simulink model "System_Modell"  (R2018a)
settings: Solver=FixedStepAuto  StartTime=0.0  StopTime=inf  FixedStep=1/f  RelTol=1e-3
values from neighbouring files (symbols this model uses):
  f = 10000    [System_Init.m]
(part 7 of 8)

== matlab function System_Modell/Motor_3/MotionSM_1/MATLAB Function ==
  data: status input double size=1; excute_signal output boolean size=1; message_to_send output double size=2; data_received input double size=2; ZZP_wait data_store_memory size=1; AP data_store_memory; ZZP data_store_memory
%data_received / message_to_send = [cmd, ZZP]
%cmd:  1...setP, 2...getP, 3...excP

function [excute_signal, message_to_send] = message_analysis(status, data_received)

global ZZP_wait
global AP
global ZZP

excute_signal = false;

cmd = data_received(1);
message_to_send = [0, 0]';

switch cmd
    case 1      % setP
        excute_signal = false;
        if ((status >= 1) && (status <= 3))
            ZZP_wait = data_received(2);
            message_to_send = [2, ZZP_wait]';   % getP
        end
        
    case 3      % excP
        excute_signal = true;
        if ((ZZP == AP) && (status == 2) && (ZZP~=ZZP_wait))
            ZZP = ZZP_wait;
        end
end
end

== matlab function System_Modell/Motor_3/MotionSM_1/Motor/MATLAB Function ==
  settings: updateMethod=DISCRETE
  data: status_Motor output boolean size=1; Motor_control_signal input double size=1; parameter input double size=4; v input double size=1; a output double size=1; direction output double size=1; AP data_store_memory; ZZP data_store_memory
function [status_Motor, a, direction]= Motor(Motor_control_signal, parameter, v)

%delta_T = parameter(1);
a_max = abs(parameter(2));
v_max = abs(parameter(3));
s0 = parameter(4);
direction = 0;
a = 0;

s_a = 0.5 * v_max * v_max / a_max;
a_bremsen = 100000;     % 100 m/s^2

global AP
global ZZP

switch Motor_control_signal
    case {-1, 0}            %Error & Off
        if v > 0
            a = -a_bremsen;
            direction = 1;
        elseif v < 0
            a = a_bremsen;
            direction = -1;
        else
            a = 0;
            direction = 0;
        end
             
    case 1                  %Init
        if (AP > 0)
            direction = s0;
            if ((ZZP - AP) < (-s_a)) && (v > (-v_max))
                a = -a_max;
            elseif ((ZZP - AP) >= (-s_a)) && (ZZP < AP) && (v < 0)
                a = a_max;
            else
                a = 0;
            end
        else
            a = 0;
            AP = 0;
        end
        
    case 2                  %Stop
        if (v > 0)
            a = -a_max;
            direction = 1;
        elseif (v < 0)
            a = a_max;
            direction = -1;
        else
            a = 0;
            direction = 0;
        end
        
    case 3                  %run
        direction = s0;
        if (s0 > 0)   %forward
            %v_control(2) = s0;
            if ((ZZP - AP) > s_a) && (v < v_max)
                a = a_max;
            elseif ((ZZP - AP) <= s_a) && (ZZP > AP) && (v > 0)
                a = -a_max;
            else
                a = 0;
            end
        end
        if (s0 < 0)    %backward
            if ((ZZP - AP) < (-s_a)) && (v > (-v_max))
                a = -a_max;
            elseif ((ZZP - AP) >= (-s_a)) && (ZZP < AP) && (v < 0)
                a = a_max;
            else
                a = 0;
            end
        end
end
        
%status_Motor: false...Stopped, true...Running
if (a == 0) && (v == 0)
    status_Motor = false;
else
    status_Motor = true;
end

end

== matlab function System_Modell/Motor_3/MotionSM_1/Motor/MATLAB Function1 ==
  settings: updateMethod=DISCRETE
  data: V output; v input; direction input double size=1; AP data_store_memory; ZZP data_store_memory
function V = v_conrol(v, direction)

global AP
global ZZP

if direction > 0
    if ((v < 0) || (AP >= ZZP))
        V = 0;
    else
        V = v;
    end
elseif direction < 0
    if v > 0 || (AP <= ZZP)
        V = 0;
    else
        V = v;
    end
else
    V = 0;
end
end

== matlab function System_Modell/Motor_3/MotionSM_1/Motor/MATLAB Function2 ==
  settings: updateMethod=DISCRETE
  data: s input; s_old input; S output; direction input double size=1; AP data_store_memory; ZZP data_store_memory
function S = s_control(s, s_old, direction)

global AP
global ZZP

if direction > 0
    if (AP + s - s_old) < ZZP
        S = s;
        AP = AP + s - s_old;
    else
        S = s_old;
        AP = ZZP;
    end
elseif direction < 0
    if (AP + s - s_old) > ZZP
        S = s;
        AP = AP + s - s_old;
    else
        S = s_old;
        AP = ZZP;
    end
else
    S = s_old;
end

end

== matlab function System_Modell/Motor_3/Schnittstelle_0/Add_to_Send_Buffer ==
  data: Send_Buffer_1 data_store_memory; Send_Buffer_2 data_store_memory; Address data_store_memory; status input; lenS_1 input; lenS_2 input; to_send_signal input; to_send_package input; Address_1 data_store_memory; Address_2 data_store_memory; Handshake_1 data_store_memory; Handshake_2 data_store_memory; Filter data_store_memory; De_1 data_store_memory; De_2 data_store_memory; De_sum_1 data_store_memory; De_sum_2 data_store_memory
% Name: add_to_Send_Buffer
% Funktionalitäten
% Handshake-Message einfügen, wenn Status==1
% Delay-caculation-Message einfügen, wenn Status==2
% Sum-Delay-caculation-Message einfügen, wemm Status==3
% Nachrichten, die der Host senden möchte, einfügen, wenn Status==4

function add_to_Send_Buffer(status, lenS_1, lenS_2, to_send_signal, to_send_package)

global Send_Buffer_1
global Send_Buffer_2
global Address
global Address_1
global Address_2
global Handshake_1
global Handshake_2
global Filter
global De_1
global De_2
global De_sum_1
global De_sum_2

switch status
    case -2                         % Error Signal einrichten
        Filter(1,7) = 1;
    case 1                          % Handshake
        if((Filter(1,1) == 0) && ~Handshake_1)              % 103 not sent yet || Handshake_1 not finish yet
            check_1 = check_X(103, Address, Send_Buffer_1);          % check if there is a 103-Message in Send_Buffer_1
            if ~check_1
                Send_Buffer_1(lenS_1:lenS_1+7) = [Address, 0, 103, zeros(1,4), 102];
                Filter(1,1) = 1;                            % to remember, if 103 ist sent
            end
        end
        if((Filter(1,2) == 0) && ~Handshake_2)
            check_2 = check_X(103, Address, Send_Buffer_2);
            if ~check_2
                Send_Buffer_2(lenS_2:lenS_2+7) = [Address, 0, 103, zeros(1,4), 102];
                Filter(1,2) = 1;
            end
        end

        
    case 2                          % Delay time caculation
        if((Filter(1,3) == 0 ) && (De_1 <= 0))              % 105 not sent || De_1 not caculated yet
            check_1 = check_X(105, Address, Send_Buffer_1);
            if ~check_1
                Send_Buffer_1(lenS_1:lenS_1+7) = [Address, Address_2, 105, zeros(1,4), 102];
                Filter(1,3) = 1;
            end
        end
        if((Filter(1,4) == 0 ) && (De_2 <= 0))
            check_2 = check_X(105, Address, Send_Buffer_2);
            if ~check_2
                Send_Buffer_2(lenS_2:lenS_2+7) = [Address, Address_1, 105, zeros(1,4), 102];
                Filter(1,4) = 1;
            end
        end
        
    case 3                          % Sum_Delay caculation
        if((Filter(1,5) == 0 ) && (De_sum_1 <= 0))          % 107 not sent || De_sum_1 not caculated yet
            check_1 = check_X(107, Address, Send_Buffer_1);
            if ~check_1
                Send_Buffer_1(lenS_1:lenS_1+7) = [Address, Address, 107, zeros(1,4), 102];
                Filter(1,5) = 1;
            end
        end
        if((Filter(1,6) == 0 ) && (De_sum_2 <= 0))
            check_2 = check_X(107, Address, Send_Buffer_2);
            if ~check_2
                Send_Buffer_2(lenS_2:lenS_2+7) = [Address, Address, 107, zeros(1,4), 102];
                Filter(1,6) = 1;
            end
        end
        
    case 4                          % normal communication
        if to_send_signal
            check_1 = check_Y(to_send_package, Send_Buffer_1);
            check_2 = check_Y(to_send_package, Send_Buffer_2);
            if ~check_1
                Send_Buffer_1(lenS_1:lenS_1+7) = [to_send_package, 102];
            end
            if ~check_2
                Send_Buffer_2(lenS_2:lenS_2+7) = [to_send_package, 102];
            end
        end
end

end

function y = check_X(CMD, adr, Data)          % y: boolean; x: double, [1x100];

x = find(Data==CMD);
y = ~isempty(x);
if y
    y = y && (Data(1,x(1)-2) == adr);
end

end

function y = check_Y(data, Data)          % y: boolean; data: double, [1x6];

x = find(Data==data(3));        % CMD
y = ~isempty(x);
if y
    for i=1:length(x)
        if(isequal(Data(x(i)-2:x(i)+3),data(1:6)))
            y = true;
            break
        else
            y = false;
        end
    end
end

end

== matlab function System_Modell/Motor_3/Schnittstelle_0/Global_Var_Length ==
  data: len_Send_Buffer_1 output double size=1; len_Send_Buffer_2 output double size=1; len_Recv_Buffer output double size=1; len_Filter output double size=1; Send_Buffer_1 data_store_memory; Send_Buffer_2 data_store_memory; Recv_Buffer data_store_memory; Filter data_store_memory
% genutzte Länge der globale Variablen berechnen

function [len_Send_Buffer_1, len_Send_Buffer_2, len_Recv_Buffer, len_Filter] = Length
global Send_Buffer_1
global Send_Buffer_2
global Recv_Buffer
global Filter

a1 = find(Send_Buffer_1==102,1);
len_Send_Buffer_1 = a1(1);
a2 = find(Send_Buffer_2==102,1);
len_Send_Buffer_2 = a2(1);

len_Recv_Buffer = min(find(Recv_Buffer==0,150))-1;
len_Filter = min(find(Filter(2:20)==0,150));

end

== matlab function System_Modell/Motor_3/Schnittstelle_0/Recv_1 ==
  data: status input double size=1; clock input double size=1; lenS_1 input; lenS_2 input; lenR input; Rx_1_signal input boolean size=1; Rx_1_data input double size=[1 100]; recv_signal_1 output boolean; recv_package_1 output double size=[1 98]; Send_Buffer_1 data_store_memory; Send_Buffer_2 data_store_memory; T_send_1 data_store_memory; T_recv_1 data_store_memory; De_1 data_store_memory; De_sum_1 data_store_memory; Address data_store_memory; Recv_Buffer data_store_memory; Address_2 data_store_memory; Address_1 data_store_memory; De_sum_2 data_store_memory; Handshake_1 data_store_memory; De_2 data_store_memory; Handshake_2 data_store_memory; T_recv_2 data_store_memory; T_send_2 data_store_memory
% Name: Rx_1

% -------------------------------------------------------------------------------------
% Funktionalitäten:
% Im Init-Prozess
%   1. Handshake durch zu führen
%       103...Handshake ask --> 104 in Send_Buffer_2 additieren
%       104...Handshake answer --> Handshake success
%   2. Delay-Zeit berechnen
%       105...Delay begin --> 106 in Send_Buffer_2 additieren
%       106...Delay end --> Delay_Zeit berechnen
%   3. Sum-Delay-Zeit berechnen
%       107, Receiver = meine Addresse --> Sum_Delay_Zeit berechnen
%       107, Receiver ~= meine Addresse --> Daten in Send_Buffer_1 additieren
% Im normalen Prozess
%   4. Receiver = meine Addresse --> in Recv_Buffer additieren
%   5. Receiver = 255 --> Broadcast --> in Recv_Buffer && Send_Buffer_1 additieren
%   6. Receiver ~= meine Addresse --> in Send_Buffer_1 additieren

% -------------------------------------------------------------------------------------
% Input && Output
% status - status of 'Schnittstelle'
% clock - simulation time
% lenS_1/len_2/lenR - meaningful length of Send_Buffer_1/Send_Buffer_2/Recv_Buffer
% Rx_1_data - from Rx_1 received data
% recv_package_1 - data to send to chart or store in Send_Buffer_1
    % in Init-process, recv_package_1 need to be sent to chart
    % in normal-process, recv_package_1 need to garther all 'to be transmmited' datablock, and store in Send_Buffer_1

function [recv_signal_1, recv_package_1] = Rx_1(status, clock,lenS_1, lenS_2, lenR, Rx_1_signal, Rx_1_data)

global Send_Buffer_1
global Send_Buffer_2
global T_send_1
global T_recv_1
global De_1
%global De_2
global De_sum_1
global Address
global Address_1
%global Address_2
global Recv_Buffer
global Handshake_1

recv_signal_1 = false;
recv_package_1 = zeros(1,98);       % one datablock = [1x7]

lenr = 1;                           % path to write data into recv_package_1

if Rx_1_signal
    a = find(Rx_1_data==102,1);
    len = a(1);
    if ~isempty(len)
        mod_ = mod(len-2,7);
        len_ = ceil((len - 2) / 7);                                 % Round toward positive infinity
    end
    
	if ((mod_ == 0) && (len_ >= 1))                             % package contains at least one datablock
        switch status
            case 1                                              % Handshake
                for i=1:len_
                    switch Rx_1_data(7*i-3)                          % Da.cmd
                        case 103                                % Handshake ask --> send answer
                            check = check_X(104, Address, Send_Buffer_2);
                            if ((Rx_1_data(7*i-5) ~= 0) && (Rx_1_data(7*i-4) == 0) && ~Handshake_1 && ~check)
                                Address_1 = Rx_1_data(7*i-5);
                                Send_Buffer_2(lenS_2:lenS_2+7) = [Address, Address_1, 104, zeros(1,4), 102];
                            end
                        case 104                                % Handshake answer --> Handshake success --> no more send
                            if ((Rx_1_data(7*i-5) ~= 0) && (Rx_1_data(7*i-4) == Address) && ~Handshake_1)
                                Address_1 = Rx_1_data(7*i-5);        % Address of the Host in the Direction_1
                                recv_package_1(lenr:lenr+6) = Rx_1_data(7*i-5:7*i+1);    % [_,_,104,_,_,_,_] = [1x7]
                                lenr = lenr + 7;
                                recv_signal_1 = true;
                            end
                    end
                end

            case 2                                              % Delay_Time_Caculation
                for j=1:len_
                    switch Rx_1_data(7*j-3)                          % Da.cmd
                        case 103                                % Handshake ask --> send answer
                            check = check_X(104, Address, Send_Buffer_2);
                            if ((Rx_1_data(7*j-5) ~= 0) && (Rx_1_data(7*j-4) == 0) && ~Handshake_1 && ~check)
                                Address_1 = Rx_1_data(7*j-5);
                                Send_Buffer_2(lenS_2:lenS_2+7) = [Address, Address_1, 104, zeros(1,4), 102];
                            end
                        case 105                                % Delay ask --> send answer
                            check = check_X(106, Address, Send_Buffer_2);
                            if (isequal(Rx_1_data(7*j-5:7*j-4),[Address_1, Address]) && Handshake_1 && ~check) % check Sender & Receiver
                                Send_Buffer_2(lenS_2:lenS_2+7) = [Address, Address_1, 106, zeros(1,4), 102];
                            end
                        case 106                                % Delay answer --> caculate the time --> no more send
                            if ((isequal(Rx_1_data(7*j-5:7*j-3),[Address_1, Address, 106])) && (De_1 <= 0) && (T_send_1 > 0))
                                T_recv_1 = clock;
                                De_1 = T_recv_1 - T_send_1;
                                T_send_1 = 0;
                                T_recv_1 = 0;
                            end
                    end
                end

            case 3                                              % Sum_Delay_Caculation
                for h=1:len_
                    switch Rx_1_data(7*h-3)
                        case 103                                % Handshake ask --> send answer
                            check = check_X(104, Address, Send_Buffer_2);
                            if ((Rx_1_data(7*h-5) ~= 0) && (Rx_1_data(7*h-4) == 0) && ~Handshake_1 && ~check)
                                Address_1 = Rx_1_data(7*h-5);
                                Send_Buffer_2(lenS_2:lenS_2+7) = [Address, Address_1, 104, zeros(1,4), 102];
                            end
                        case 105                                % Delay ask --> send answer
                            check = check_X(106, Address, Send_Buffer_2);
                            if (isequal(Rx_1_data(7*h-5:7*h-4),[Address_1, Address]) && Handshake_1 && ~check) % check Sender & Receiver
                                Send_Buffer_2(lenS_2:lenS_2+7) = [Address, 0, 106, zeros(1,4), 102];
                            end   
                        case 107
                            if (isequal(Rx_1_data(7*h-5:7*h-4),[Address, Address]) && (De_sum_1 <= De_1) && (T_send_1 > 0))                   % Sum_Delay --> caculate the time --> no more send
                                T_recv_1 = clock;
                                De_sum_1 = T_recv_1 - T_send_1;
                                T_send_1 = 0;
                                T_recv_1 = 0;
                            elseif ((isequal(Rx_1_data(7*h-5),Rx_1_data(7*h-4))) && (Rx_1_data(7*h-5) ~= Address))
                                check = check_Y(Rx_1_data(7*h-5:7*h), recv_package_1) || check_Y(Rx_1_data(7*h-5:7*h), Send_Buffer_1);
                                if ~check
                                    recv_package_1(lenr:lenr+6) = Rx_1_data(7*h-5:7*h+1)';
                                    lenr = lenr + 7;
                                end
                            end
                    end
                end
                Send_Buffer_1(lenS_1:lenS_1+lenr-1) = [recv_package_1(1:lenr-1),102];           % 前提：lenS更新速度比当前更新快

            case 4                                               % normal communication between all Hosts
                for k=1:len_
                    switch Rx_1_data(7*k-3)
                        case 103                                % Handshake ask --> send answer
                            check = check_X(104, Address, Send_Buffer_2);
                            if ((Rx_1_data(7*k-5) ~= 0) && (Rx_1_data(7*k-4) == 0) && ~Handshake_1 && ~check)
                                Address_1 = Rx_1_data(7*k-5);
                                Send_Buffer_2(lenS_2:lenS_2+7) = [Address, Address_1, 104, zeros(1,4), 102];
                            end
                        case 105                                % Delay ask --> send answer
                            check = check_X(106, Address, Send_Buffer_2);
                            if (isequal(Rx_1_data(7*k-5:7*k-4),[Address_1, Address]) && Handshake_1 && ~check) % check Sender & Receiver
                                Send_Buffer_2(lenS_2:lenS_2+7) = [Address, 0, 106, zeros(1,4), 102];
                            end
                        case 107
                            if ((isequal(Rx_1_data(7*k-5),Rx_1_data(7*k-4))) && (Rx_1_data(7*k-5) ~= Address))
                                check = check_Y(Rx_1_data(7*k-5:7*k), recv_package_1) || check_Y(Rx_1_data(7*k-5:7*k), Send_Buffer_1);
                                if ~check
                                    recv_package_1(lenr:lenr+6) = Rx_1_data(7*k-5:7*k+1)';
                                    lenr = lenr + 7;
                                end
                            end
                        otherwise
                            if ((Rx_1_data(7*k-5) ~= Address) && (Rx_1_data(7*k-4) == Address))   % Datablock sent to me --> store in Recv_Buffer
                                check = check_Y(Rx_1_data(7*k-5:7*k), Recv_Buffer');
                                if ~check
                                    Recv_Buffer(lenR+1,:) = Rx_1_data(7*k-5:7*k+1);
                                end
                            elseif ((Rx_1_data(7*k-5) ~=Address) && (Rx_1_data(7*k-4) == 255))    % Datablock is as a Broadcast --> store in Recv_Buffer && Send_Buffer_1
                                check = check_Y(Rx_1_data(7*k-5:7*k), Recv_Buffer');
                                if ~check
                                    Recv_Buffer(lenR+1,:) = Rx_1_data(7*k-5:7*k+1);
                                end
                                check = check_Y(Rx_1_data(7*k-5:7*k), recv_package_1) || check_Y(Rx_1_data(7*k-5:7*k), Send_Buffer_1);
                                if ~check
                                    recv_package_1(lenr:lenr+6) = Rx_1_data(7*k-5:7*k+1)';
                                    lenr = lenr + 7;
                                end
                            elseif ((Rx_1_data(7*k-4) ~= Address) && (Rx_1_data(7*k-4) ~= 255))   % Datablock not sent to me --> to transmmit --> store in Send_Buffer_1
                                check = check_Y(Rx_1_data(7*k-5:7*k), recv_package_1) || check_Y(Rx_1_data(7*k-5:7*k), Send_Buffer_1);
                                if ~check
                                    recv_package_1(lenr:lenr+6) = Rx_1_data(7*k-5:7*k+1)';
                                    lenr = lenr + 7;
                                end
                            end
                    end
                end
                Send_Buffer_1(lenS_1:lenS_1+lenr-1) = [recv_package_1(1:lenr-1),102];
        end
	elseif mod_ ~= 0
        fprintf("Eroor: Package length not avalueable!");
	end
end

end

% check_X: to check if Data contains a Datablock with CMD and adr
function y = check_X(CMD, adr, Data)          % y: boolean; x: double, [1x100];

x = find(Data==CMD);
y = (~isempty(x));

if y
    y = y && (Data(1,x(1)-2) == adr);
end

end

% check_Y: to check if Data contains data
function y = check_Y(data, Data)          % y: boolean; data: double, [1x6];

x = find(Data==data(3));
y = (~isempty(x));
if y
    for i=1:length(x)
        if(isequal(Data(x(i)-2:x(i)+3),data))
            y = true;
            break
        else
            y = false;
        end
    end
end

end

== matlab function System_Modell/Motor_3/Schnittstelle_0/Recv_2 ==
  data: status input double size=1; clock input double size=1; lenS_1 input; lenS_2 input; lenR input; Rx_2_signal input boolean size=1; Rx_2_data input double size=[1 100]; recv_signal_2 output boolean; recv_package_2 output double size=[1 98]; Send_Buffer_1 data_store_memory; Send_Buffer_2 data_store_memory; T_send_1 data_store_memory; T_recv_1 data_store_memory; De_1 data_store_memory; De_sum_1 data_store_memory; Address data_store_memory; Recv_Buffer data_store_memory; Address_2 data_store_memory; Address_1 data_store_memory; De_sum_2 data_store_memory; Handshake_1 data_store_memory; De_2 data_store_memory; Handshake_2 data_store_memory; T_recv_2 data_store_memory; T_send_2 data_store_memory
% Name: Rx_2

% -------------------------------------------------------------------------------------
% Funktionalitäten:
% Im Init-Prozess
%   1. Handshake durch zu führen
%       103...Handshake ask --> 104 in Send_Buffer_1 additieren
%       104...Handshake answer --> Handshake success
%   2. Delay-Zeit berechnen
%       105...Delay begin --> 106 in Send_Buffer_1 additieren
%       106...Delay end --> Delay_Zeit berechnen
%   3. Sum-Delay-Zeit berechnen
%       107, Receiver = meine Addresse --> Sum_Delay_Zeit berechnen
%       107, Receiver ~= meine Addresse --> Daten in Send_Buffer_2 additieren
% Im normalen Prozess
%   4. Receiver = meine Addresse --> in Recv_Buffer additieren
%   5. Receiver = 255 --> Broadcast --> in Recv_Buffer && Send_Buffer_2 additieren
%   6. Receiver ~= meine Addresse --> in Send_Buffer_2 additieren

% -------------------------------------------------------------------------------------
% Input && Output
% status - status of 'Schnittstelle'
% clock - simulation time
% lenS_2/len_1/lenR - meaningful length of Send_Buffer_2/Send_Buffer_1/Recv_Buffer
% Rx_2_data - from Rx_2 received data
% recv_package_2 - data to send to chart or store in Send_Buffer_2
    % in Init-process, recv_package_2 need to be sent to chart
    % in normal-process, recv_package_2 need to garther all 'to be transmmited' datablock, and store in Send_Buffer_2

function [recv_signal_2, recv_package_2] = Rx_2(status, clock,lenS_1, lenS_2, lenR, Rx_2_signal, Rx_2_data)

global Send_Buffer_2
global Send_Buffer_1
global T_send_2
global T_recv_2
global De_2
%global De_1
global De_sum_2
global Address
global Address_2
%global Address_1
global Recv_Buffer
global Handshake_2

recv_signal_2 = false;
recv_package_2 = zeros(1,98);       % one datablock = [1x7]

lenr = 1;                           % path to write data into recv_package_2

if Rx_2_signal
    a = find(Rx_2_data==102,1);
    len = a(1);
    if ~isempty(len)
        mod_ = mod(len-2,7);
        len_ = ceil((len - 2) / 7);                                 % Round toward positive infinity
    end
    
	if ((mod_ == 0) && (len_ >= 1))                             % package contains at least one datablock
        switch status
            case 1                                              % Handshake
                for i=1:len_
                    switch Rx_2_data(7*i-3)                          % Da.cmd
                        case 103                                % Handshake ask --> send answer
                            check = check_X(104, Address, Send_Buffer_1);
                            if ((Rx_2_data(7*i-5) ~= 0) && (Rx_2_data(7*i-4) == 0) && ~Handshake_2 && ~check)
                                Address_2 = Rx_2_data(7*i-5);
                                Send_Buffer_1(lenS_1:lenS_1+7) = [Address, Address_2, 104, zeros(1,4), 102];
                            end
                        case 104                                % Handshake answer --> Handshake success --> no more send
                            if ((Rx_2_data(7*i-5) ~= 0) && (Rx_2_data(7*i-4) == Address) && ~Handshake_2)
                                Address_2 = Rx_2_data(7*i-5);        % Address of the Host in the Direction_2
                                recv_package_2(lenr:lenr+6) = Rx_2_data(7*i-5:7*i+1);    % [_,_,104,_,_,_,_] = [1x7]
                                lenr = lenr + 7;
                                recv_signal_2 = true;
                            end
                    end
                end

            case 2                                              % Delay_Time_Caculation
                for j=1:len_
                    switch Rx_2_data(7*j-3)                          % Da.cmd
                        case 103                                % Handshake ask --> send answer
                            check = check_X(104, Address, Send_Buffer_1);
                            if ((Rx_2_data(7*j-5) ~= 0) && (Rx_2_data(7*j-4) == 0) && ~Handshake_2 && ~check)
                                Address_2 = Rx_2_data(7*j-5);
                                Send_Buffer_1(lenS_1:lenS_1+7) = [Address, Address_2, 104, zeros(1,4), 102];
                            end
                        case 105                                % Delay ask --> send answer
                            check = check_X(106, Address, Send_Buffer_1);
                            if (isequal(Rx_2_data(7*j-5:7*j-4),[Address_2, Address]) && Handshake_2 && ~check) % check Sender & Receiver
                                Send_Buffer_1(lenS_1:lenS_1+7) = [Address, Address_2, 106, zeros(1,4), 102];
                            end
                        case 106                                % Delay answer --> caculate the time --> no more send
                            if ((isequal(Rx_2_data(7*j-5:7*j-3),[Address_2, Address, 106])) && (De_2 <= 0) && (T_send_2 > 0))
                                T_recv_2 = clock;
                                De_2 = T_recv_2 - T_send_2;
                                T_send_2 = 0;
                                T_recv_2 = 0;
                            end
                    end
                end

            case 3                                              % Sum_Delay_Caculation
                for h=1:len_
                    switch Rx_2_data(7*h-3)
                        case 103                                % Handshake ask --> send answer
                            check = check_X(104, Address, Send_Buffer_1);
                            if ((Rx_2_data(7*h-5) ~= 0) && (Rx_2_data(7*h-4) == 0) && ~Handshake_2 && ~check)
                                Address_2 = Rx_2_data(7*h-5);
                                Send_Buffer_1(lenS_1:lenS_1+7) = [Address, Address_2, 104, zeros(1,4), 102];
                            end
                        case 105                                % Delay ask --> send answer
                            check = check_X(106, Address, Send_Buffer_1);
                            if (isequal(Rx_2_data(7*h-5:7*h-4),[Address_2, Address]) && Handshake_2 && ~check) % check Sender & Receiver
                                Send_Buffer_1(lenS_1:lenS_1+7) = [Address, Address_2, 106, zeros(1,4), 102];
                            end   
                        case 107
                            if (isequal(Rx_2_data(7*h-5:7*h-4),[Address, Address]) && (De_sum_2 <= De_2) && (T_send_2 > 0))                   % Sum_Delay --> caculate the time --> no more send
                                T_recv_2 = clock;
                                De_sum_2 = T_recv_2 - T_send_2;
                                T_send_2 = 0;
                                T_recv_2 = 0;
                            elseif ((isequal(Rx_2_data(7*h-5),Rx_2_data(7*h-4))) && (Rx_2_data(7*h-5) ~= Address))
                                check = check_Y(Rx_2_data(7*h-5:7*h), recv_package_2) || check_Y(Rx_2_data(7*h-5:7*h), Send_Buffer_2);
                                if ~check
                                    recv_package_2(lenr:lenr+6) = Rx_2_data(7*h-5:7*h+1)';
                                    lenr = lenr + 7;
                                end
                            end
                    end
                end
                Send_Buffer_2(lenS_2:lenS_2+lenr-1) = [recv_package_2(1:lenr-1),102];           % 前提：lenS更新速度比当前更新快

            case 4                                               % normal communication between all Hosts
                for k=1:len_
                    switch Rx_2_data(7*k-3)
                        case 103                                % Handshake ask --> send answer
                            check = check_X(104, Address, Send_Buffer_1);
                            if ((Rx_2_data(7*k-5) ~= 0) && (Rx_2_data(7*k-4) == 0) && ~Handshake_2 && ~check)
                                Address_2 = Rx_2_data(7*k-5);
                                Send_Buffer_1(lenS_1:lenS_1+7) = [Address, Address_2, 104, zeros(1,4), 102];
                            end
                        case 105                                % Delay ask --> send answer
                            check = check_X(106, Address, Send_Buffer_1);
                            if (isequal(Rx_2_data(7*k-5:7*k-4),[Address_2, Address]) && Handshake_2 && ~check) % check Sender & Receiver
                                Send_Buffer_1(lenS_1:lenS_1+7) = [Address, 0, 106, zeros(1,4), 102];
                            end
                        case 107
                            if ((isequal(Rx_2_data(7*k-5),Rx_2_data(7*k-4))) && (Rx_2_data(7*k-5) ~= Address))
                                check = check_Y(Rx_2_data(7*k-5:7*k), recv_package_2) || check_Y(Rx_2_data(7*k-5:7*k), Send_Buffer_2);
                                if ~check
                                    recv_package_2(lenr:lenr+6) = Rx_2_data(7*k-5:7*k+1)';
                                    lenr = lenr + 7;
                                end
                            end
                        otherwise
                            if ((Rx_2_data(7*k-5) ~= Address) && (Rx_2_data(7*k-4) == Address))   % Datablock sent to me --> store in Recv_Buffer
                                check = check_Y(Rx_2_data(7*k-5:7*k), Recv_Buffer');
                                if ~check
                                    Recv_Buffer(lenR+1,:) = Rx_2_data(7*k-5:7*k+1);
                                end
                            elseif ((Rx_2_data(7*k-5) ~=Address) && (Rx_2_data(7*k-4) == 255))    % Datablock is as a Broadcast --> store in Recv_Buffer && Send_Buffer_2
                                check = check_Y(Rx_2_data(7*k-5:7*k), Recv_Buffer');
                                if ~check
                                    Recv_Buffer(lenR+1,:) = Rx_2_data(7*k-5:7*k+1);
                                end
                                check = check_Y(Rx_2_data(7*k-5:7*k), recv_package_2) || check_Y(Rx_2_data(7*k-5:7*k), Send_Buffer_2);
                                if ~check
                                    recv_package_2(lenr:lenr+6) = Rx_2_data(7*k-5:7*k+1)';
                                    lenr = lenr + 7;
                                end
                            elseif ((Rx_2_data(7*k-4) ~= Address) && (Rx_2_data(7*k-4) ~= 255))   % Datablock not sent to me --> to transmmit --> store in Send_Buffer_2
                                check = check_Y(Rx_2_data(7*k-5:7*k), recv_package_2) || check_Y(Rx_2_data(7*k-5:7*k), Send_Buffer_2);
                                if ~check
                                    recv_package_2(lenr:lenr+6) = Rx_2_data(7*k-5:7*k+1)';
                                    lenr = lenr + 7;
                                end
                            end
                    end
                end
                Send_Buffer_2(lenS_2:lenS_2+lenr-1) = [recv_package_2(1:lenr-1),102];
        end
	elseif mod_ ~= 0
        fprintf("Eroor: Package length not avalueable!");
	end
end

end

% check_X: to check if Data contains a Datablock with CMD and adr
function y = check_X(CMD, adr, Data)          % y: boolean; x: double, [1x100];

x = find(Data==CMD);
y = (~isempty(x));

if y
    y = y && (Data(1,x(1)-2) == adr);
end

end

% check_Y: to check if Data contains data
function y = check_Y(data, Data)          % y: boolean; data: double, [1x6];

x = find(Data==data(3));
y = (~isempty(x));
if y
    for i=1:length(x)
        if(isequal(Data(x(i)-2:x(i)+3),data))
            y = true;
            break
        else
            y = false;
        end
    end
end

end

== matlab function System_Modell/Motor_1/Schnittstelle_0/Send_Telegram/Send_Telegram_2 ==
  data: status input double size=1; clock input double; lenS_2 input; impulse input boolean size=1; Tx_2_signal output boolean size=1; Tx_2_data output double size=[1,100]; send_2_old input boolean size=1; T_send_1 data_store_memory; T_send_2 data_store_memory; Send_Buffer_1 data_store_memory; Send_Buffer_2 data_store_memory; De_1 data_store_memory; De_2 data_store_memory; De_sum_1 data_store_memory; De_sum_2 data_store_memory; Address data_store_memory
% Name: send_telegram
% Funktionalität:
% Datenpacket in Send_Buffer_2 und Send_Buffer2 zyklisch transferieren.
% Die Zykluszeit lautet 10ms

function [Tx_2_signal, Tx_2_data] = send_telegram_2(status, clock, lenS_2, impulse, send_2_old)

global Send_Buffer_2
global De_2
global De_sum_2
global T_send_2
global Address

timer_2 = 0;

if send_2_old
    % The Send_Signal lasts for only one period. Then it need to be shut down.
    Tx_2_signal = false;
    Tx_2_data = [101,102,zeros(1,98)];
else
    % No Error + send-signal already shut down + Impulse-Signal --> OK! Let's send the telegram!
    h1 = ceil((lenS_2 - 2) / 7);
    if ((status > 0) && (~send_2_old) && impulse && (h1 > 0))
        % Before send, we need check if we need to do something else. For example: 'start the Timer' or 'caculate a new De in each datablock'
        switch status
            case 2                                              % Delay time caculation
                if ~isempty(find(Send_Buffer_2==105,1))                     % check if there is a 105-cmd in Send_Buffer,if so, timer need to be started
                    timer_2 = 1;
                end

            case 3                                              % Sum_Delay caculation
                for i1=1:h1
                    if isequal([Send_Buffer_2(7*i1-5:7*i1-3),De_sum_2],[Address,Address,107,0])     % check if there is a 107-cmd in Send_Buffer
                        timer_2 = 1;
                        break
                    end
                end

            case 4
                for i1=1:h1                                                    % recaculate the Delay time for each datablock
                    Send_Buffer_2(7*i1+1) = Send_Buffer_2(7*i1+1) + De_2;
                end
        end
        
        % Now we can send the telegram!!
        Tx_2_data = Send_Buffer_2;                                  % send data
        Tx_2_signal = true;
        
        % remember the send-time if necessary
        if timer_2 == 1
            T_send_2 = clock;
        end
        
        % clear the data in Send_Buffer after sending
        Send_Buffer_2 = [101,102,zeros(1,98)];

    else
        Tx_2_signal = false;
        Tx_2_data = [101,102,zeros(1,98)];
    end
end

end

== matlab function System_Modell/Kabel1_3/Telegramm_Stethoskop ==
  data: Signal output; Data output; signal input; data input
function [Signal, Data]= Telegramm_Stethoskop(signal, data)

if signal
    D = data
else
    D = zeros(1,100);
end

Signal = signal;
Data = data;

end

== matlab function System_Modell/ZP_Mananger/Schnittstelle_1/Send_Telegram/Send_Telegram1 ==
  data: status input double size=1; clock input double; lenS_2 input; impulse input boolean size=1; Tx_2_signal output boolean size=1; Tx_2_data output double size=[1,100]; send_2_old input boolean size=1; T_send_1 data_store_memory; T_send_2 data_store_memory; Send_Buffer_1 data_store_memory; Send_Buffer_2 data_store_memory; De_1 data_store_memory; De_2 data_store_memory; De_sum_1 data_store_memory; De_sum_2 data_store_memory; Address data_store_memory
% Name: send_telegram
% Funktionalität:
% Datenpacket in Send_Buffer_2 und Send_Buffer2 zyklisch transferieren.
% Die Zykluszeit lautet 10ms

function [Tx_2_signal, Tx_2_data] = send_telegram(status, clock, lenS_2, impulse, send_2_old)

global Send_Buffer_2
global De_2
global De_sum_2
global T_send_2
global Address

timer_2 = 0;

if send_2_old
    % The Send_Signal lasts for only one period. Then it need to be shut down.
    Tx_2_signal = false;
    Tx_2_data = [101,102,zeros(1,98)];
else
    % No Error + send-signal already shut down + Impulse-Signal --> OK! Let's send the telegram!
    h1 = ceil((lenS_2 - 2) / 7);
    if ((status > 0) && (~send_2_old) && impulse && (h1 > 0))
        % Before send, we need check if we need to do something else. For example: 'start the Timer' or 'caculate a new De in each datablock'
        switch status
            case 2                                              % Delay time caculation
                if ~isempty(find(Send_Buffer_2==105,1))                     % check if there is a 105-cmd in Send_Buffer,if so, timer need to be started
                    timer_2 = 1;
                end

            case 3                                              % Sum_Delay caculation
                for i1=1:h1
                    if isequal([Send_Buffer_2(7*i1-5:7*i1-3),De_sum_2],[Address,Address,107,0])     % check if there is a 107-cmd in Send_Buffer
                        timer_2 = 1;
                        break
                    end
                end

            case 4
                for i1=1:h1                                                    % recaculate the Delay time for each datablock
                    Send_Buffer_2(7*i1+1) = Send_Buffer_2(7*i1+1) + De_2;
                end
        end
        
        % Now we can send the telegram!!
        Tx_2_data = Send_Buffer_2;                                  % send data
        Tx_2_signal = true;
        
        % remember the send-time if necessary
        if timer_2 == 1
            T_send_2 = clock;
        end
        
        % clear the data in Send_Buffer after sending
        Send_Buffer_2 = [101,102,zeros(1,98)];

    else
        Tx_2_signal = false;
        Tx_2_data = [101,102,zeros(1,98)];
    end
end

end

== matlab function System_Modell/Motor_3/Schnittstelle_0/Send_Telegram/Send_Done_1 ==
  data: wait2send_sgn input; send_done_1 output; wait2send_pkg input; Tx_1_sgn input; Tx_1_data input
function send_done_1 = Send_Done_1(wait2send_sgn, wait2send_pkg, Tx_1_sgn, Tx_1_data)

if (wait2send_sgn && Tx_1_sgn)
    X = find(Tx_1_data==115,1);
    if ~isempty(X)
        if isequal(Tx_1_data(1, X(1)-2:X(1)+4), wait2send_pkg)
            send_done_1 = true;
        else
            send_done_1 = false;
        end
    else
        send_done_1 =false;
    end
else
    send_done_1 = false;
end

end

== matlab function System_Modell/Motor_3/Schnittstelle_0/Send_Telegram/Send_Done_2 ==
  data: wait2send_sgn input; send_done_2 output; wait2send_pkg input; Tx_2_sgn input; Tx_2_data input
function send_done_2 = Send_Done_2(wait2send_sgn, wait2send_pkg, Tx_2_sgn, Tx_2_data)

if (wait2send_sgn && Tx_2_sgn)
    X = find(Tx_2_data==115,1);
    if ~isempty(X)
        if isequal(Tx_2_data(1, X(1)-2:X(1)+4), wait2send_pkg)
            send_done_2 = true;
        else
            send_done_2 = false;
        end
    else
        send_done_2 =false;
    end
else
    send_done_2 = false;
end

end

== matlab function System_Modell/Motor_3/Schnittstelle_0/Send_Telegram/Send_Telegram_1 ==
  data: status input double size=1; clock input double; lenS_1 input; impulse input boolean size=1; Tx_1_signal output boolean size=1; Tx_1_data output double size=[1,100]; send_1_old input boolean size=1; T_send_1 data_store_memory; T_send_2 data_store_memory; Send_Buffer_1 data_store_memory; Send_Buffer_2 data_store_memory; De_1 data_store_memory; De_2 data_store_memory; De_sum_1 data_store_memory; De_sum_2 data_store_memory; Address data_store_memory
% Name: send_telegram
% Funktionalität:
% Datenpacket in Send_Buffer_1 und Send_Buffer2 zyklisch transferieren.
% Die Zykluszeit lautet 10ms

function [Tx_1_signal, Tx_1_data] = send_telegram_1(status, clock, lenS_1, impulse, send_1_old)

global Send_Buffer_1
global De_1
global De_sum_1
global T_send_1
global Address

timer_1 = 0;

if send_1_old
    % The Send_Signal lasts for only one period. Then it need to be shut down.
    Tx_1_signal = false;
    Tx_1_data = [101,102,zeros(1,98)];
else
    % No Error + send-signal already shut down + Impulse-Signal --> OK! Let's send the telegram!
    h1 = ceil((lenS_1 - 2) / 7);
    if ((status > 0) && (~send_1_old) && impulse && (h1 > 0))
        % Before send, we need check if we need to do something else. For example: 'start the Timer' or 'caculate a new De in each datablock'
        switch status
            case 2                                              % Delay time caculation
                if ~isempty(find(Send_Buffer_1==105,1))                     % check if there is a 105-cmd in Send_Buffer,if so, timer need to be started
                    timer_1 = 1;
                end

            case 3                                              % Sum_Delay caculation
                for i1=1:h1
                    if isequal([Send_Buffer_1(7*i1-5:7*i1-3),De_sum_1],[Address,Address,107,0])     % check if there is a 107-cmd in Send_Buffer
                        timer_1 = 1;
                        break
                    end
                end

            case 4
                for i1=1:h1                                                    % recaculate the Delay time for each datablock
                    Send_Buffer_1(7*i1+1) = Send_Buffer_1(7*i1+1) + De_1;
                end
        end
        
        % Now we can send the telegram!!
        Tx_1_data = Send_Buffer_1;                                  % send data
        Tx_1_signal = true;
        
        % remember the send-time if necessary
        if timer_1 == 1
            T_send_1 = clock;
        end
        
        % clear the data in Send_Buffer after sending
        Send_Buffer_1 = [101,102,zeros(1,98)];

    else
        Tx_1_signal = false;
        Tx_1_data = [101,102,zeros(1,98)];
    end
end

end

== matlab function System_Modell/Motor_3/Schnittstelle_0/Send_Telegram/Send_Telegram_2 ==
  data: status input double size=1; clock input double; lenS_2 input; impulse input boolean size=1; Tx_2_signal output boolean size=1; Tx_2_data output double size=[1,100]; send_2_old input boolean size=1; T_send_1 data_store_memory; T_send_2 data_store_memory; Send_Buffer_1 data_store_memory; Send_Buffer_2 data_store_memory; De_1 data_store_memory; De_2 data_store_memory; De_sum_1 data_store_memory; De_sum_2 data_store_memory; Address data_store_memory
% Name: send_telegram
% Funktionalität:
% Datenpacket in Send_Buffer_2 und Send_Buffer2 zyklisch transferieren.
% Die Zykluszeit lautet 10ms

function [Tx_2_signal, Tx_2_data] = send_telegram_2(status, clock, lenS_2, impulse, send_2_old)

global Send_Buffer_2
global De_2
global De_sum_2
global T_send_2
global Address

timer_2 = 0;

if send_2_old
    % The Send_Signal lasts for only one period. Then it need to be shut down.
    Tx_2_signal = false;
    Tx_2_data = [101,102,zeros(1,98)];
else
    % No Error + send-signal already shut down + Impulse-Signal --> OK! Let's send the telegram!
    h1 = ceil((lenS_2 - 2) / 7);
    if ((status > 0) && (~send_2_old) && impulse && (h1 > 0))
        % Before send, we need check if we need to do something else. For example: 'start the Timer' or 'caculate a new De in each datablock'
        switch status
            case 2                                              % Delay time caculation
                if ~isempty(find(Send_Buffer_2==105,1))                     % check if there is a 105-cmd in Send_Buffer,if so, timer need to be started
                    timer_2 = 1;
                end

            case 3                                              % Sum_Delay caculation
                for i1=1:h1
                    if isequal([Send_Buffer_2(7*i1-5:7*i1-3),De_sum_2],[Address,Address,107,0])     % check if there is a 107-cmd in Send_Buffer
                        timer_2 = 1;
                        break
                    end
                end

            case 4
                for i1=1:h1                                                    % recaculate the Delay time for each datablock
                    Send_Buffer_2(7*i1+1) = Send_Buffer_2(7*i1+1) + De_2;
                end
        end
        
        % Now we can send the telegram!!
        Tx_2_data = Send_Buffer_2;                                  % send data
        Tx_2_signal = true;
        
        % remember the send-time if necessary
        if timer_2 == 1
            T_send_2 = clock;
        end
        
        % clear the data in Send_Buffer after sending
        Send_Buffer_2 = [101,102,zeros(1,98)];

    else
        Tx_2_signal = false;
        Tx_2_data = [101,102,zeros(1,98)];
    end
end

end

== matlab function System_Modell/Motor_1/Schnittstelle_0/Send_Telegram/Send_Done_1 ==
  data: wait2send_sgn input; send_done_1 output; wait2send_pkg input; Tx_1_sgn input; Tx_1_data input
function send_done_1 = Send_Done_1(wait2send_sgn, wait2send_pkg, Tx_1_sgn, Tx_1_data)

if (wait2send_sgn && Tx_1_sgn)
    X = find(Tx_1_data==115,1);
    if ~isempty(X)
        if isequal(Tx_1_data(1, X(1)-2:X(1)+4), wait2send_pkg)
            send_done_1 = true;
        else
            send_done_1 = false;
        end
    else
        send_done_1 =false;
    end
else
    send_done_1 = false;
end

end

== matlab function System_Modell/Motor_1/Schnittstelle_0/Send_Telegram/Send_Done_2 ==
  data: wait2send_sgn input; send_done_2 output; wait2send_pkg input; Tx_2_sgn input; Tx_2_data input
function send_done_2 = Send_Done_2(wait2send_sgn, wait2send_pkg, Tx_2_sgn, Tx_2_data)

if (wait2send_sgn && Tx_2_sgn)
    X = find(Tx_2_data==115,1);
    if ~isempty(X)
        if isequal(Tx_2_data(1, X(1)-2:X(1)+4), wait2send_pkg)
            send_done_2 = true;
        else
            send_done_2 = false;
        end
    else
        send_done_2 =false;
    end
else
    send_done_2 = false;
end

end
